simulink model "quick_start_qbot_platform"  (R2023a)
settings: Solver=ode1  StartTime=0.0  StopTime=Inf  FixedStep=1/60  RelTol=1e-3
PostLoadFcn:
  | qlabs_setup
model workspace (MAT data in the model file):
  Sig = Simulink.Signal
  Sig.DataType = 'auto'
  Sig.Dimensions = -1
  Sig.DimensionsMode = 'auto'
  Sig.Complexity = 'auto'
  Sig.SampleTime = -1
  Sig.SamplingMode = 'auto'
  downCamStepSize = Simulink.Parameter
  downCamStepSize.Value = Simulink.data.Expression
  downCamStepSize.Value.ExpressionString = "qc_get_step_size*ceil(1/30/qc_get_step_size)"
  downCamStepSize.DataType = 'auto'
  downCamStepSize.Complexity = 'real'
  downCamStepSize.Dimensions = -1
  lidarStepSize = Simulink.Parameter
  lidarStepSize.Value = Simulink.data.Expression
  lidarStepSize.Value.ExpressionString = "qc_get_step_size*ceil(1/5/qc_get_step_size)"
  lidarStepSize.DataType = 'auto'
  lidarStepSize.Complexity = 'real'
  lidarStepSize.Dimensions = -1
  mainStepSize = Simulink.Parameter
  mainStepSize.Value = Simulink.data.Expression
  mainStepSize.Value.ExpressionString = "qc_get_step_size"
  mainStepSize.DataType = 'auto'
  mainStepSize.Complexity = 'real'
  mainStepSize.Dimensions = -1
  mode = Simulink.Parameter
  mode.Value = 1
  mode.Description = '0 - education speeds via wheel speed commands
    | 1 - education speeds via body speed commands
    | 2 - research speeds via wheel speed commands
    | 3 - research speeds via body speed commands'
  mode.DataType = 'auto'
  mode.Complexity = 'real'
  mode.Dimensions = [1 1]
  realSenseStepSize = Simulink.Parameter
  realSenseStepSize.Value = Simulink.data.Expression
  realSenseStepSize.Value.ExpressionString = "qc_get_step_size*ceil(1/30/qc_get_step_size)"
  realSenseStepSize.DataType = 'auto'
  realSenseStepSize.Complexity = 'real'
  realSenseStepSize.Dimensions = -1
undefined symbols (not defined in the file or in its folder): gcbh, JPEG, Point, qc_get_step_size, Video3D, video_display_show
libraries: quarc_library x31
settings Model: SimulationMode=external  ExtModeTrigDuration=10000  Creator=mbohra  LastModifiedBy=mbohra
settings DebuggingCC: UnderspecifiedInitializationDetection=Classic  MergeDetectMultiDrivingBlocksExec=none
settings ModelReferenceCC: PropagateSignalLabelsOutOfModel=off

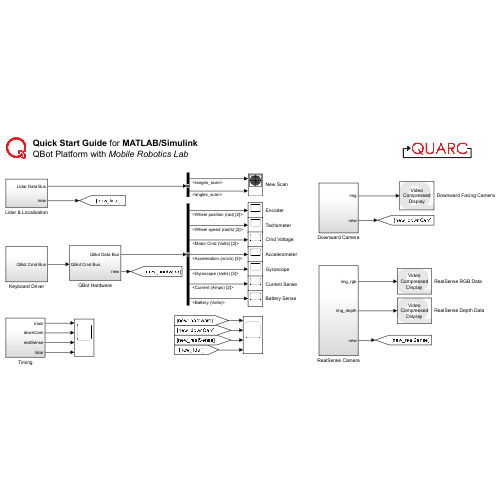
[thumbnail: Simulink's stored preview of the top-level diagram]
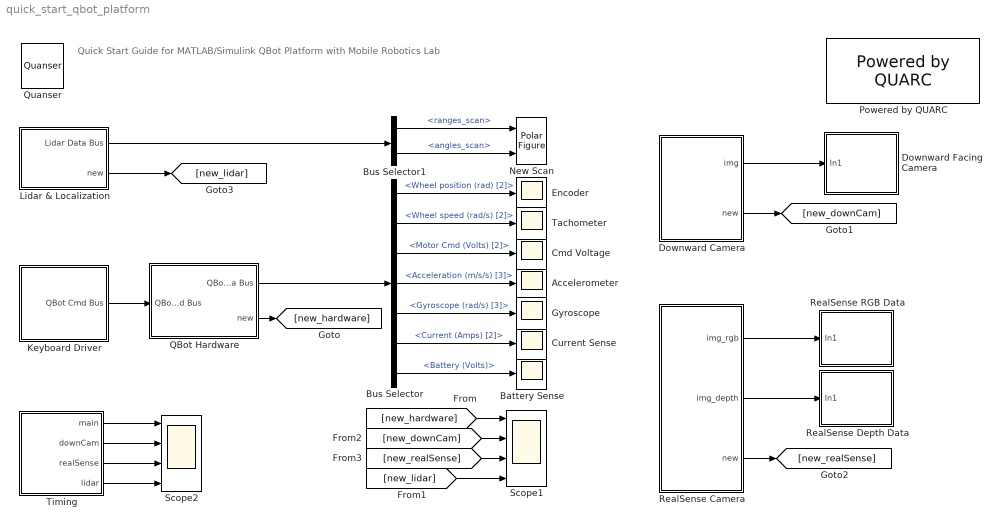
== system quick_start_qbot_platform ==
  note: Quick Start Guide for MATLAB/Simulink
      | QBot Platform with Mobile Robotics Lab
  Accelerometer : Scope
  Battery Sense : Scope
  Bus Selector : BusSelector  OutputSignals=Wheel position (rad) [2],Wheel speed (rad/s) [2],Motor Cmd (Volts) [2],Acceleration (m/s/s) [3],Gyroscope (rad/s) [3],Current (Amps) [2],Battery (Volts)
  Bus Selector1 : BusSelector  OutputSignals=ranges_scan,angles_scan
  Cmd Voltage : Scope
  Current Sense : Scope
  Downward Camera : Subsystem
  Downward Facing Camera : Subsystem  LoadFcn=set_param(gcbh, 'UserData', gcb);  StartFcn=video_display_show([gcb, '/Video Display'], 'add', gcb);  mask(Video Compressed Display){algorithm=JPEG, quality=50, sample_time=-1, use_hardware=on}
      mask prompts: algorithm "Compression algorithm:"; quality "Compression quality (0-100):"; sample_time "Sample time (seconds):"; use_hardware "Use hardware acceleration for video display"
      mask help: Displays a video stream on the host, using compression to minimize bandwidth.
      mask init:
      | qc_set_display('Video\nCompressed\nDisplay');
      settings: UndoDeleteFcn=set_param(gcbh, 'UserData', gcb);  OpenFcn=video_display_show([gcb, '/Video Display'], 'show', gcb);  PreDeleteFcn=video_display_show([gcb, '/Video Display'], 'delete');
      settings: CopyFcn=|
      | set_param(gcbh, 'UserData', gcb);
      | set_param(gcbh, 'LinkStatus', 'none');
      settings: NameChangeFcn=|
      | video_display_show([get_param(gcbh, 'UserData'), '/Video Display'], 'rename', [gcb, '/Video Display']);
      | video_display_show([gcb, '/Video Display'], 'add', gcb);
      | set_param(gcbh, 'UserData', gcb);
      mask Help: web(qc_get_block_help_path(gcb));
      mask TypeOptions algorithm: Image Compress/algorithm
      mask TypeOptions quality: Image Compress/quality
      mask TypeOptions sample_time: Video Display/sample_time
      mask TypeOptions use_hardware: Video Display/use_hardware
      mask Display:
      | patch([0.98591 0.98591 0.62618 0.59072 0.56147   0.536   0.536  0.5441 0.56912 0.59207 0.60881 0.62276 0.63527 0.64364  0.6485  0.6485 0.64706 0.64499 0.63662 0.62411 0.61232 0.59837 0.58307 0.56147   0.536   0.536  0.5441  0.5747 0.60953 0.63662 0.67001  0.7034 0.72851 0.75425 0.77927 0.80294 0.82454 0.84119 0.85865 0.87395 0.88574 0.89339  0.8969 0.89969 0.89969 0.89267  0.8816 0.87044 0.85649  0.8384 0.81824 0.80294 0.78764 0.77513 0.76676 0.75776 0.76397 0.77513 0.79178 0.80987 0.82796 0.84326 0.86207 0.98528],[0.18689 0.05522 0.05522 0.05171 0.05171    0.05 0.18338 0.18338 0.19148 0.20435 0.22298 0.24863 0.28589 0.33125 0.38138 0.55139 0.59801 0.63761 0.68189 0.72149 0.74939 0.76694 0.77855 0.79367 0.79952 0.92768 0.92768 0.92768 0.92417 0.92066 0.91364  0.9032 0.89384 0.88106 0.86594 0.85073 0.82634 0.80537 0.77855 0.74363 0.70403 0.65858 0.61079 0.59099 0.41513 0.37202 0.31847 0.29048 0.25556 0.23342  0.2102 0.19382 0.18221 0.17285 0.16943 0.16124  0.1589 0.16241 0.16709 0.17168  0.1787 0.18221 0.18689 0.18689],[0.9,0.90,0.91])
      | patch([0.536 0.52601 0.46823 0.44528 0.41603 0.39101 0.35555 0.33116 0.31451 0.29291  0.2804 0.26717 0.25322 0.23999 0.22406 0.20732 0.19337 0.17528 0.15935 0.14396 0.13217 0.11759 0.10922 0.10085 0.09671 0.09392 0.09041 0.08906 0.08906 0.09464  0.0995 0.10778 0.11894 0.13145 0.14675 0.16349 0.17672 0.19409 0.20732 0.22406 0.23999 0.26159 0.27833 0.29849 0.31793 0.33602 0.35411 0.37085 0.39245 0.41603   0.536   0.536 0.53159 0.46409   0.446 0.42026 0.39587 0.37571 0.36113 0.34925 0.34088 0.33809 0.33809 0.34088 0.34583 0.35627 0.36392 0.38129 0.39587 0.41117 0.42719 0.44672  0.4676 0.48353 0.48353 0.52394   0.536],[0.05 0.04829 0.04712 0.04712 0.04829 0.05063 0.05405 0.05873 0.06107 0.06692 0.07043 0.07619 0.08087 0.08672 0.09482 0.10652 0.11696 0.13325  0.1508 0.17168 0.19499 0.22415 0.25439 0.28472 0.31379 0.35456 0.38489 0.41513 0.58055 0.63878 0.68774 0.72149 0.75641 0.78089 0.80537 0.82859 0.84029 0.85658 0.86594 0.87404  0.8834 0.89267 0.90086 0.90788 0.91247 0.91832 0.92066   0.923 0.92651 0.92768 0.92768 0.79952 0.79952 0.79952 0.79718 0.78899 0.77153 0.75056 0.72149 0.68072 0.62249  0.5549 0.41396 0.37085 0.33242 0.28121 0.25205 0.22181 0.20552 0.19499 0.18572 0.18221 0.17753 0.17636 0.17753  0.1787  0.1787],[0.9,0.90,0.91])
      | disp('Video\nCompressed\nDisplay');
  Encoder : Scope
  Gyroscope : Scope
  Keyboard Driver : Subsystem
  Lidar & Localization : Subsystem
  New Scan : quarc_library/Sinks/Figures/Polar Figure  figure_mode=Use figure window  figure_tag=figure1  axes_tag=axes1  plot_mode=Frame-based  minimum_rho=0  maximum_rho=4  minimum_theta=0  maximum_theta=360  zero_location=top  direction=counterclockwise  buffer_size=1  update_rate=1  sample_time=-1  initial_position="1340   385   433   389"  initial_visibility=off  line1_style=None  line1_width=0.5  line1_color=[0 0.4470 0.7410]  marker1=Point (.)  marker1_size=6  marker1_edge_color=[0 0.447059 0.741176]  marker1_face_color=[0 0.447059 0.741176]  line2_style=Solid line (-)  line2_width=0.5  line2_color=[0.85098 0.32549 0.0980392]  marker2=None  marker2_size=6  marker2_edge_color=[0.85098 0.32549 0.0980392]  marker2_face_color=[0.85098 0.32549 0.0980392]  line3_style=Solid line (-)  line3_width=0.5  line3_color=[0.929412 0.694118 0.12549]  marker3=None  marker3_size=6  marker3_edge_color=[0.929412 0.694118 0.12549]  marker3_face_color=[0.929412 0.694118 0.12549]  line4_style=Solid line (-)  line4_width=0.5  line4_color=[0.494118 0.184314 0.556863]  marker4=None  marker4_size=6  marker4_edge_color=[0.494118 0.184314 0.556863]  marker4_face_color=[0.494118 0.184314 0.556863]  line5_style=Solid line (-)  line5_width=0.5  line5_color=[0.466667 0.67451 0.188235]  marker5=None  marker5_size=6  marker5_edge_color=[0.466667 0.67451 0.188235]  marker5_face_color=[0.466667 0.67451 0.188235]
      settings: SourceProductName=QUARC Targets
  Powered by QUARC : quarc_library/Logos/Powered by QUARC
  QBot Hardware : Subsystem
  Quanser : quarc_library/Logos/Quanser
  RealSense Camera : Subsystem
  RealSense Depth Data : Subsystem  LoadFcn=set_param(gcbh, 'UserData', gcb);  StartFcn=video_display_show([gcb, '/Video Display'], 'add', gcb);  mask(Video Compressed Display){algorithm=JPEG, quality=50, sample_time=-1, use_hardware=on}
      mask prompts: algorithm "Compression algorithm:"; quality "Compression quality (0-100):"; sample_time "Sample time (seconds):"; use_hardware "Use hardware acceleration for video display"
      mask help: Displays a video stream on the host, using compression to minimize bandwidth.
      mask init:
      | qc_set_display('Video\nCompressed\nDisplay');
      settings: UndoDeleteFcn=set_param(gcbh, 'UserData', gcb);  OpenFcn=video_display_show([gcb, '/Video Display'], 'show', gcb);  PreDeleteFcn=video_display_show([gcb, '/Video Display'], 'delete');
      settings: CopyFcn=|
      | set_param(gcbh, 'UserData', gcb);
      | set_param(gcbh, 'LinkStatus', 'none');
      settings: NameChangeFcn=|
      | video_display_show([get_param(gcbh, 'UserData'), '/Video Display'], 'rename', [gcb, '/Video Display']);
      | video_display_show([gcb, '/Video Display'], 'add', gcb);
      | set_param(gcbh, 'UserData', gcb);
      mask Help: web(qc_get_block_help_path(gcb));
      mask TypeOptions algorithm: Image Compress/algorithm
      mask TypeOptions quality: Image Compress/quality
      mask TypeOptions sample_time: Video Display/sample_time
      mask TypeOptions use_hardware: Video Display/use_hardware
      mask Display:
      | patch([0.98591 0.98591 0.62618 0.59072 0.56147   0.536   0.536  0.5441 0.56912 0.59207 0.60881 0.62276 0.63527 0.64364  0.6485  0.6485 0.64706 0.64499 0.63662 0.62411 0.61232 0.59837 0.58307 0.56147   0.536   0.536  0.5441  0.5747 0.60953 0.63662 0.67001  0.7034 0.72851 0.75425 0.77927 0.80294 0.82454 0.84119 0.85865 0.87395 0.88574 0.89339  0.8969 0.89969 0.89969 0.89267  0.8816 0.87044 0.85649  0.8384 0.81824 0.80294 0.78764 0.77513 0.76676 0.75776 0.76397 0.77513 0.79178 0.80987 0.82796 0.84326 0.86207 0.98528],[0.18689 0.05522 0.05522 0.05171 0.05171    0.05 0.18338 0.18338 0.19148 0.20435 0.22298 0.24863 0.28589 0.33125 0.38138 0.55139 0.59801 0.63761 0.68189 0.72149 0.74939 0.76694 0.77855 0.79367 0.79952 0.92768 0.92768 0.92768 0.92417 0.92066 0.91364  0.9032 0.89384 0.88106 0.86594 0.85073 0.82634 0.80537 0.77855 0.74363 0.70403 0.65858 0.61079 0.59099 0.41513 0.37202 0.31847 0.29048 0.25556 0.23342  0.2102 0.19382 0.18221 0.17285 0.16943 0.16124  0.1589 0.16241 0.16709 0.17168  0.1787 0.18221 0.18689 0.18689],[0.9,0.90,0.91])
      | patch([0.536 0.52601 0.46823 0.44528 0.41603 0.39101 0.35555 0.33116 0.31451 0.29291  0.2804 0.26717 0.25322 0.23999 0.22406 0.20732 0.19337 0.17528 0.15935 0.14396 0.13217 0.11759 0.10922 0.10085 0.09671 0.09392 0.09041 0.08906 0.08906 0.09464  0.0995 0.10778 0.11894 0.13145 0.14675 0.16349 0.17672 0.19409 0.20732 0.22406 0.23999 0.26159 0.27833 0.29849 0.31793 0.33602 0.35411 0.37085 0.39245 0.41603   0.536   0.536 0.53159 0.46409   0.446 0.42026 0.39587 0.37571 0.36113 0.34925 0.34088 0.33809 0.33809 0.34088 0.34583 0.35627 0.36392 0.38129 0.39587 0.41117 0.42719 0.44672  0.4676 0.48353 0.48353 0.52394   0.536],[0.05 0.04829 0.04712 0.04712 0.04829 0.05063 0.05405 0.05873 0.06107 0.06692 0.07043 0.07619 0.08087 0.08672 0.09482 0.10652 0.11696 0.13325  0.1508 0.17168 0.19499 0.22415 0.25439 0.28472 0.31379 0.35456 0.38489 0.41513 0.58055 0.63878 0.68774 0.72149 0.75641 0.78089 0.80537 0.82859 0.84029 0.85658 0.86594 0.87404  0.8834 0.89267 0.90086 0.90788 0.91247 0.91832 0.92066   0.923 0.92651 0.92768 0.92768 0.79952 0.79952 0.79952 0.79718 0.78899 0.77153 0.75056 0.72149 0.68072 0.62249  0.5549 0.41396 0.37085 0.33242 0.28121 0.25205 0.22181 0.20552 0.19499 0.18572 0.18221 0.17753 0.17636 0.17753  0.1787  0.1787],[0.9,0.90,0.91])
      | disp('Video\nCompressed\nDisplay');
  RealSense RGB Data : Subsystem  LoadFcn=set_param(gcbh, 'UserData', gcb);  StartFcn=video_display_show([gcb, '/Video Display'], 'add', gcb);  mask(Video Compressed Display){algorithm=JPEG, quality=50, sample_time=-1, use_hardware=on}
      mask prompts: algorithm "Compression algorithm:"; quality "Compression quality (0-100):"; sample_time "Sample time (seconds):"; use_hardware "Use hardware acceleration for video display"
      mask help: Displays a video stream on the host, using compression to minimize bandwidth.
      mask init:
      | qc_set_display('Video\nCompressed\nDisplay');
      settings: UndoDeleteFcn=set_param(gcbh, 'UserData', gcb);  OpenFcn=video_display_show([gcb, '/Video Display'], 'show', gcb);  PreDeleteFcn=video_display_show([gcb, '/Video Display'], 'delete');
      settings: CopyFcn=|
      | set_param(gcbh, 'UserData', gcb);
      | set_param(gcbh, 'LinkStatus', 'none');
      settings: NameChangeFcn=|
      | video_display_show([get_param(gcbh, 'UserData'), '/Video Display'], 'rename', [gcb, '/Video Display']);
      | video_display_show([gcb, '/Video Display'], 'add', gcb);
      | set_param(gcbh, 'UserData', gcb);
      mask Help: web(qc_get_block_help_path(gcb));
      mask TypeOptions algorithm: Image Compress/algorithm
      mask TypeOptions quality: Image Compress/quality
      mask TypeOptions sample_time: Video Display/sample_time
      mask TypeOptions use_hardware: Video Display/use_hardware
      mask Display:
      | patch([0.98591 0.98591 0.62618 0.59072 0.56147   0.536   0.536  0.5441 0.56912 0.59207 0.60881 0.62276 0.63527 0.64364  0.6485  0.6485 0.64706 0.64499 0.63662 0.62411 0.61232 0.59837 0.58307 0.56147   0.536   0.536  0.5441  0.5747 0.60953 0.63662 0.67001  0.7034 0.72851 0.75425 0.77927 0.80294 0.82454 0.84119 0.85865 0.87395 0.88574 0.89339  0.8969 0.89969 0.89969 0.89267  0.8816 0.87044 0.85649  0.8384 0.81824 0.80294 0.78764 0.77513 0.76676 0.75776 0.76397 0.77513 0.79178 0.80987 0.82796 0.84326 0.86207 0.98528],[0.18689 0.05522 0.05522 0.05171 0.05171    0.05 0.18338 0.18338 0.19148 0.20435 0.22298 0.24863 0.28589 0.33125 0.38138 0.55139 0.59801 0.63761 0.68189 0.72149 0.74939 0.76694 0.77855 0.79367 0.79952 0.92768 0.92768 0.92768 0.92417 0.92066 0.91364  0.9032 0.89384 0.88106 0.86594 0.85073 0.82634 0.80537 0.77855 0.74363 0.70403 0.65858 0.61079 0.59099 0.41513 0.37202 0.31847 0.29048 0.25556 0.23342  0.2102 0.19382 0.18221 0.17285 0.16943 0.16124  0.1589 0.16241 0.16709 0.17168  0.1787 0.18221 0.18689 0.18689],[0.9,0.90,0.91])
      | patch([0.536 0.52601 0.46823 0.44528 0.41603 0.39101 0.35555 0.33116 0.31451 0.29291  0.2804 0.26717 0.25322 0.23999 0.22406 0.20732 0.19337 0.17528 0.15935 0.14396 0.13217 0.11759 0.10922 0.10085 0.09671 0.09392 0.09041 0.08906 0.08906 0.09464  0.0995 0.10778 0.11894 0.13145 0.14675 0.16349 0.17672 0.19409 0.20732 0.22406 0.23999 0.26159 0.27833 0.29849 0.31793 0.33602 0.35411 0.37085 0.39245 0.41603   0.536   0.536 0.53159 0.46409   0.446 0.42026 0.39587 0.37571 0.36113 0.34925 0.34088 0.33809 0.33809 0.34088 0.34583 0.35627 0.36392 0.38129 0.39587 0.41117 0.42719 0.44672  0.4676 0.48353 0.48353 0.52394   0.536],[0.05 0.04829 0.04712 0.04712 0.04829 0.05063 0.05405 0.05873 0.06107 0.06692 0.07043 0.07619 0.08087 0.08672 0.09482 0.10652 0.11696 0.13325  0.1508 0.17168 0.19499 0.22415 0.25439 0.28472 0.31379 0.35456 0.38489 0.41513 0.58055 0.63878 0.68774 0.72149 0.75641 0.78089 0.80537 0.82859 0.84029 0.85658 0.86594 0.87404  0.8834 0.89267 0.90086 0.90788 0.91247 0.91832 0.92066   0.923 0.92651 0.92768 0.92768 0.79952 0.79952 0.79952 0.79718 0.78899 0.77153 0.75056 0.72149 0.68072 0.62249  0.5549 0.41396 0.37085 0.33242 0.28121 0.25205 0.22181 0.20552 0.19499 0.18572 0.18221 0.17753 0.17636 0.17753  0.1787  0.1787],[0.9,0.90,0.91])
      | disp('Video\nCompressed\nDisplay');
  Scope1 : Scope  NumInputPorts=4
  Scope2 : Scope  NumInputPorts=4
  Tachometer : Scope
  Timing : Subsystem
  wires:
  Timing/1(main) -> Scope2/1
  Timing/2(downCam) -> Scope2/2
  Timing/3(realSense) -> Scope2/3
  Timing/4(lidar) -> Scope2/4
  Lidar & Localization/1(Lidar Data Bus) -> Bus Selector1/1
  QBot Hardware/1(QBot Data Bus) -> Bus Selector/1
  QBot Hardware/2(new) -> [new_hardware]
  Lidar & Localization/2(new) -> [new_lidar]
  Downward Camera/2(new) -> [new_downCam]
  RealSense Camera/3(new) -> [new_realSense]
  [new_hardware] -> Scope1/1
  [new_realSense] -> Scope1/3
  [new_lidar] -> Scope1/4
  [new_downCam] -> Scope1/2
  Bus Selector/1 -> Encoder/1  "<Wheel position (rad) [2]>"
  Bus Selector/3 -> Cmd Voltage/1  "<Motor Cmd (Volts) [2]>"
  Bus Selector/4 -> Accelerometer/1  "<Acceleration (m/s/s) [3]>"
  Bus Selector/6 -> Current Sense/1  "<Current (Amps) [2]>"
  Bus Selector/2 -> Tachometer/1  "<Wheel speed (rad/s) [2]>"
  Bus Selector/5 -> Gyroscope/1  "<Gyroscope (rad/s) [3]>"
  Bus Selector/7 -> Battery Sense/1  "<Battery (Volts)>"
  Bus Selector1/1 -> New Scan/1  "<ranges_scan>"
  Bus Selector1/2 -> New Scan/2  "<angles_scan>"
  Downward Camera/1(img) -> Downward Facing Camera/1(In1)
  RealSense Camera/2(img_depth) -> RealSense Depth Data/1(In1)
  RealSense Camera/1(img_rgb) -> RealSense RGB Data/1(In1)
  Keyboard Driver/1(QBot Cmd Bus) -> QBot Hardware/1(QBot Cmd Bus)

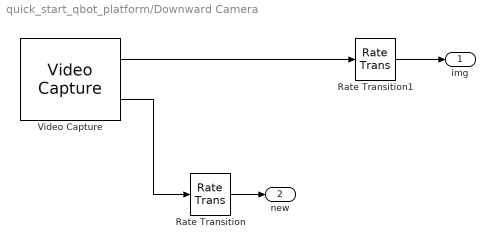
== system quick_start_qbot_platform/Downward Camera ==
  Rate Transition : RateTransition
  Rate Transition1 : RateTransition  OutPortSampleTime=downCamStepSize*4
  Video Capture : quarc_library/Multimedia/Video Capture  source=device  device=0@tcpip://localhost:18915  filename=sample_movie.mov  value=[0 0; 0 0]  resolution=640 x 400  width=640  height=400  output_format=MATLAB greyscale (HxW)  data_type=uint8  sample_time=downCamStepSize  brightness_override=off  brightness=50.0  contrast_override=off  contrast=50.0  hue_override=off  hue=50.0  saturation_override=off  saturation=50.0  sharpness_override=off  sharpness=50.0  gamma_override=off  gamma=50.0  coloreffect_override=off  coloreffect=None  whitebalance_override=off  whitebalance=50.0  backlightcompensation_override=off  backlightcompensation=0.0  gain_override=on  gain=27.0  pan_override=off  pan=50.0  tilt_override=off  tilt=50.0  roll_override=off  roll=50.0  zoom_override=off  zoom=0.0  exposure_override=on  exposure=60.0  iris_override=off  iris=50.0  mirror_override=off  mirror=None  focus_override=off  focus=0.0
      settings: SourceProductName=QUARC Targets
  img : Outport
  new : Outport  Port=2
  wires:
  Video Capture/2 -> Rate Transition/1
  Video Capture/1 -> Rate Transition1/1
  Rate Transition/1 -> new/1
  Rate Transition1/1 -> img/1

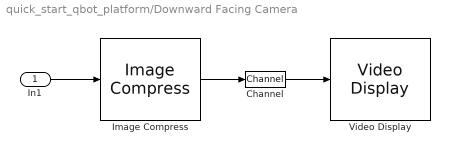
== system quick_start_qbot_platform/Downward Facing Camera ==
  In1 : Inport
  Channel : quarc_library/Signal Routing/Channel  channel=0  buffer_size=1
  Image Compress : quarc_library/Image Processing/Generic/Image Compress  algorithm=JPEG  source=Internal dialog parameter  quality=quality  output_dim=-1
  Video Display : quarc_library/Multimedia/Video Display  Tag=quick_start_qbot_platform_t/Downward Facing Camera/Video Display  sample_time=sample_time  use_hardware=on
  wires:
  Image Compress/1 -> Channel/1
  In1/1 -> Image Compress/1
  Channel/1 -> Video Display/1

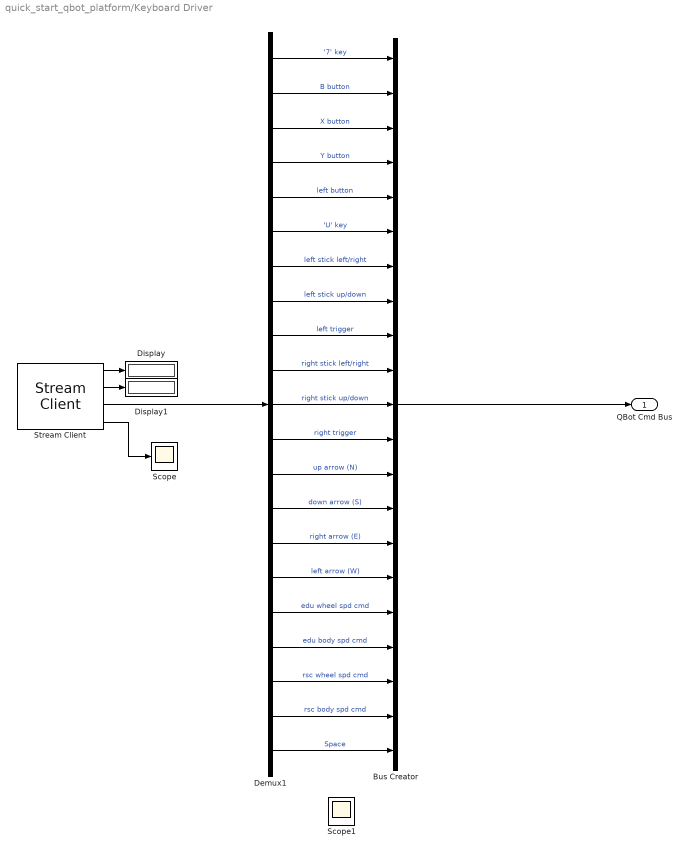
== system quick_start_qbot_platform/Keyboard Driver ==
  Bus Creator : BusCreator  Inputs=21
  Demux1 : Demux  Outputs=[1 1 1 1 1 1 1 1 1 1 1 1 1 1 1 1 2 2 2 2 1]
  Display : Display
  Display1 : Display
  Scope : Scope
  Scope1 : Scope
  Stream Client : quarc_library/Communications/Basic/Stream Client  uri_source=Specify via dialog (do not evaluate)  uri=tcpip://localhost:18889?nagle='off'  send_buffer_size=1460  receive_buffer_size=1460  byte_order=little endian (Intel - LSB first)  optimization=Minimum latency  send_options=Do not send data  receive_options=Receive most recent data  default_value=zeros(25,1)  sample_time=qc_get_step_size  active=on  implementation=Use blocking I/O in a separate thread  send_fifo_size=1000  receive_fifo_size=1000  send_priority=0  receive_priority=0  send_dimensions=off  receive_dimensions=off  max_dimensions=-1  data_type=Inherited via back propagation  type_expr=BusObject
      settings: AttributesFormatString="\"tcpip://localhost:18889?nagle='off'\""
  QBot Cmd Bus : Outport
  wires:
  Bus Creator/1 -> QBot Cmd Bus/1
  Stream Client/3 -> Demux1/1
  Demux1/1 -> Bus Creator/1  "'7' key"
  Demux1/2 -> Bus Creator/2  "B button"
  Demux1/3 -> Bus Creator/3  "X button"
  Demux1/4 -> Bus Creator/4  "Y button"
  Demux1/5 -> Bus Creator/5  "left button"
  Demux1/6 -> Bus Creator/6  "'U' key"
  Demux1/7 -> Bus Creator/7  "left stick left/right"
  Demux1/8 -> Bus Creator/8  "left stick up/down"
  Demux1/9 -> Bus Creator/9  "left trigger"
  Demux1/10 -> Bus Creator/10  "right stick left/right"
  Demux1/11 -> Bus Creator/11  "right stick up/down"
  Demux1/12 -> Bus Creator/12  "right trigger"
  Demux1/13 -> Bus Creator/13  "up arrow (N)"
  Demux1/14 -> Bus Creator/14  "down arrow (S)"
  Demux1/15 -> Bus Creator/15  "right arrow (E)"
  Demux1/16 -> Bus Creator/16  "left arrow (W)"
  Demux1/17 -> Bus Creator/17  "edu wheel spd cmd"
  Demux1/18 -> Bus Creator/18  "edu body spd cmd"
  Demux1/19 -> Bus Creator/19  "rsc wheel spd cmd"
  Demux1/20 -> Bus Creator/20  "rsc body spd cmd"
  Demux1/21 -> Bus Creator/21  "Space"
  Stream Client/1 -> Display/1
  Stream Client/2 -> Display1/1
  Stream Client/4 -> Scope/1

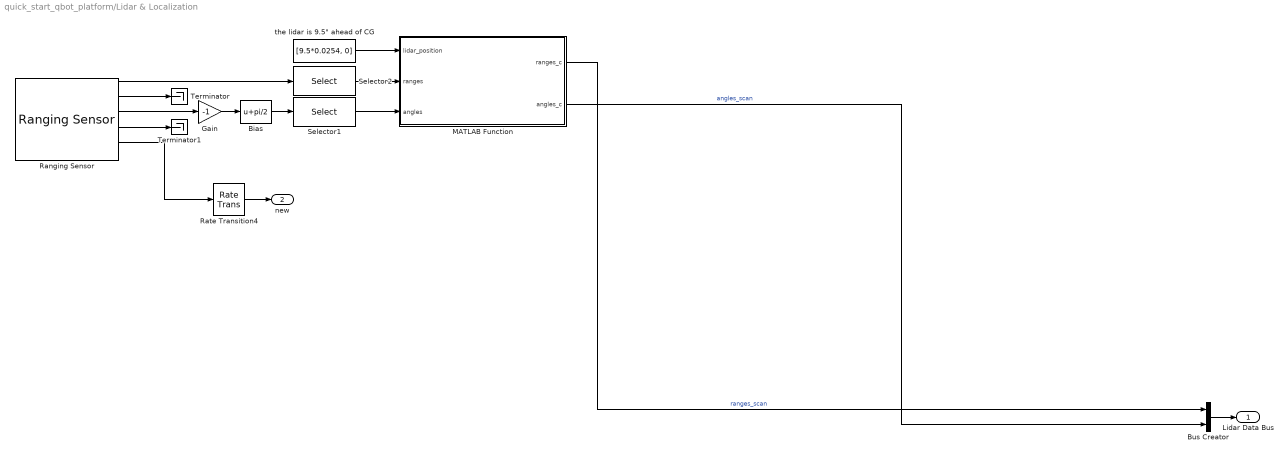
== system quick_start_qbot_platform/Lidar & Localization ==
  Bias : Bias  Bias=pi/2  SaturateOnIntegerOverflow=off
  Bus Creator : BusCreator  Inputs=2
  Gain : Gain  Gain=-1
  MATLAB Function : MATLAB Function  TreatAsAtomicUnit=on
  Ranging Sensor : quarc_library/Devices/Third-Party/Sensors/Ranging Sensor  sensor_type=Leishen M10P LIDAR  uri=tcpip://localhost:18918  ranging_distance=Short  timing_budget=0.033  measurement_period=0.0005  output_mode=Fixed-size output  samples_per_revolution=1680  max_distance=0.050  max_angle=5  sample_time=lidarStepSize  show_versions=off  active=on
      settings: SourceProductName=QUARC Targets
  Rate Transition4 : RateTransition
  Selector1 : Selector  InputPortWidth=1680  IndexOptions=Index vector (dialog)  Indices=[1:4:1677]  OutputSizes=1
  Selector2 : Selector  InputPortWidth=1680  IndexOptions=Index vector (dialog)  Indices=[1:4:1677]  OutputSizes=1
  Terminator : Terminator
  Terminator1 : Terminator
  "the lidar is 9.5\" ahead of CG" : Constant  Value=[9.5*0.0254, 0]  SampleTime=lidarStepSize
  Lidar Data Bus : Outport
  new : Outport  Port=2
  wires:
  Ranging Sensor/5 -> Rate Transition4/1
  Rate Transition4/1 -> new/1
  Selector1/1 -> MATLAB Function/3(angles)
  Selector2/1 -> MATLAB Function/2(ranges)
  "the lidar is 9.5\" ahead of CG"/1 -> MATLAB Function/1(lidar_position)
  Bias/1 -> Selector1/1
  Ranging Sensor/2 -> Terminator/1
  Ranging Sensor/4 -> Terminator1/1
  Gain/1 -> Bias/1
  Ranging Sensor/3 -> Gain/1
  Ranging Sensor/1 -> Selector2/1
  MATLAB Function/1(ranges_c) -> Bus Creator/1  "ranges_scan"
  MATLAB Function/2(angles_c) -> Bus Creator/2  "angles_scan"
  Bus Creator/1 -> Lidar Data Bus/1

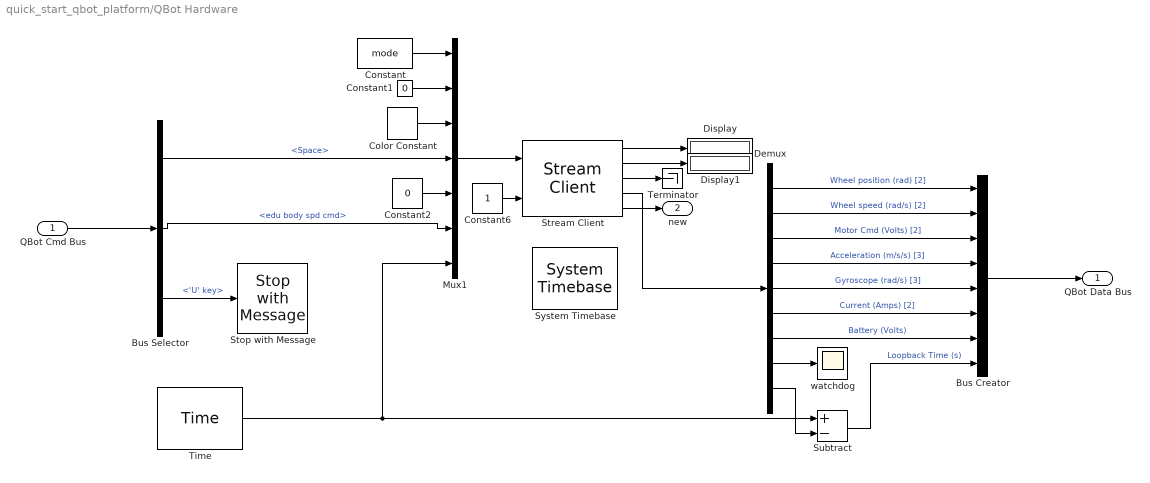
== system quick_start_qbot_platform/QBot Hardware ==
  QBot Cmd Bus : Inport
  Bus Creator : BusCreator  Inputs=8
  Bus Selector : BusSelector  OutputSignals=Space,edu body spd cmd,'U' key
  Color Constant : quarc_library/Sources/Signals/Color Constant  color=[0 1 1]
      settings: SourceProductName=QUARC Targets
  Constant : Constant  Value=mode
  Constant1 : Constant  Value=0
  Constant2 : Constant  Value=0
  Constant6 : Constant
  Demux : Demux  Outputs=[2 2 2 3 3 2 1 1 1]
  Display : Display
  Display1 : Display
  Mux1 : Mux  Inputs=7
  Stop with Message : quarc_library/Sinks/Error Handling/Stop with Message  message_type=Fixed error message  message_icon=Information  message=Operator: Emergency Stop
  Stream Client : quarc_library/Communications/Basic/Stream Client  uri_source=Specify via dialog (do not evaluate)  uri=tcpip://localhost:18888  send_buffer_size=1460  receive_buffer_size=1460  byte_order=little endian (Intel - LSB first)  optimization=Minimum latency  send_options=Send most recent data  receive_options=Receive most recent data  default_value=zeros(17,1)  sample_time=qc_get_step_size  active=on  implementation=Use blocking I/O in a separate thread  send_fifo_size=1000  receive_fifo_size=1000  send_priority=0  receive_priority=0  send_dimensions=off  receive_dimensions=off  max_dimensions=-1  data_type=Inherited via back propagation  type_expr=BusObject
      settings: AttributesFormatString="\"tcpip://localhost:18888\""
  Subtract : Sum  Inputs=+-
  System Timebase : quarc_library/Advanced/Timing/System Timebase  stop_on_overrun=off
      settings: SourceProductName=QUARC Targets
  Terminator : Terminator
  Time : quarc_library/Sources/Time/Time  time_source=Wall clock  sample_time=qc_get_step_size
  watchdog : Scope
  QBot Data Bus : Outport
  new : Outport  Port=2
  wires:
  Demux/2 -> Bus Creator/2  "Wheel speed (rad/s) [2]"
  Constant/1 -> Mux1/1
  Stream Client/3 -> Terminator/1
  Stream Client/1 -> Display/1
  Constant6/1 -> Stream Client/2
  Stream Client/2 -> Display1/1
  Color Constant/1 -> Mux1/3
  Constant1/1 -> Mux1/2
  Demux/3 -> Bus Creator/3  "Motor Cmd (Volts) [2]"
  Mux1/1 -> Stream Client/1
  Stream Client/4 -> Demux/1
  Demux/1 -> Bus Creator/1  "Wheel position (rad) [2]"
  Stream Client/5 -> new/1
  Demux/7 -> Bus Creator/7  "Battery (Volts)"
  Demux/5 -> Bus Creator/5  "Gyroscope (rad/s) [3]"
  Demux/6 -> Bus Creator/6  "Current (Amps) [2]"
  Demux/9 -> Subtract/2
  Constant2/1 -> Mux1/5
  Demux/4 -> Bus Creator/4  "Acceleration (m/s/s) [3]"
  Time/1 -> Subtract/1, Mux1/7
  Bus Creator/1 -> QBot Data Bus/1
  Subtract/1 -> Bus Creator/8  "Loopback Time (s)"
  Demux/8 -> watchdog/1
  QBot Cmd Bus/1 -> Bus Selector/1
  Bus Selector/3 -> Stop with Message/1  "<'U' key>"
  Bus Selector/2 -> Mux1/6  "<edu body spd cmd>"
  Bus Selector/1 -> Mux1/4  "<Space>"

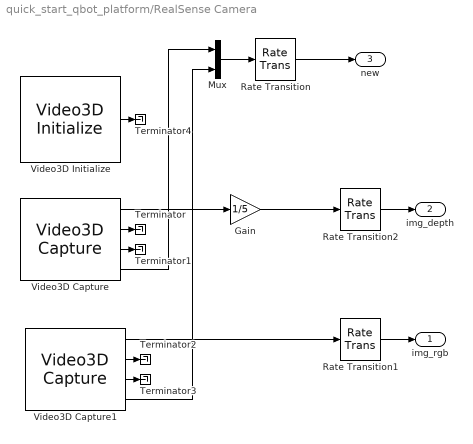
== system quick_start_qbot_platform/RealSense Camera ==
  Gain : Gain  Gain=1/5
  Mux : Mux  Inputs=2
  Rate Transition : RateTransition
  Rate Transition1 : RateTransition  OutPortSampleTime=realSenseStepSize*2
  Rate Transition2 : RateTransition  OutPortSampleTime=realSenseStepSize*2
  Terminator{,1..4} (5 alike) : Terminator
  Video3D Capture : quarc_library/Multimedia/Video3D Capture  object_name=Video3D-1  stream_type=Depth  stream_index=0  resolution=640 x 480  width=640  height=480  output_format=Distance in meters (HxW)  data_type=single  sample_time=realSenseStepSize  camera_intrinsics=off  depth_scale=off  brightness_override=off  brightness=50.0  contrast_override=off  contrast=50.0  hue_override=off  hue=50.0  saturation_override=off  saturation=50.0  sharpness_override=off  sharpness=50.0  gamma_override=off  gamma=50.0  gain_override=off  gain=50.0  backlightcompensation_override=off  backlightcompensation=50.0  whitebalance_override=Automatic white balance  whitebalance=50.0  exposure_override=Automatic exposure  exposure=30.0  emitter=Enable laser emitter  preset=Do not set camera presets
  Video3D Capture1 : quarc_library/Multimedia/Video3D Capture  object_name=Video3D-1  stream_type=RGB  stream_index=0  resolution=640 x 480  width=640  height=480  output_format=MATLAB RGB (HxWx3)  data_type=uint8  sample_time=realSenseStepSize  camera_intrinsics=off  depth_scale=off  brightness_override=off  brightness=50.0  contrast_override=off  contrast=50.0  hue_override=off  hue=50.0  saturation_override=off  saturation=50.0  sharpness_override=off  sharpness=50.0  gamma_override=off  gamma=50.0  gain_override=off  gain=50.0  backlightcompensation_override=off  backlightcompensation=50.0  whitebalance_override=Automatic white balance  whitebalance=50.0  exposure_override=Automatic exposure  exposure=30.0  emitter=Enable laser emitter  preset=Do not set camera presets
  Video3D Initialize : quarc_library/Multimedia/Video3D Initialize  object_name=Video3D-1  source=Device  identifier=0@tcpip://localhost:18917  file=sample.bag  sample_time=qc_get_step_size *2  active=on
  img_rgb : Outport
  img_depth : Outport  Port=2
  new : Outport  Port=3
  wires:
  Video3D Capture1/1 -> Rate Transition1/1
  Mux/1 -> Rate Transition/1
  Video3D Capture/4 -> Mux/1
  Video3D Capture1/4 -> Mux/2
  Video3D Capture/2 -> Terminator/1
  Video3D Capture/3 -> Terminator1/1
  Video3D Capture1/2 -> Terminator2/1
  Video3D Capture1/3 -> Terminator3/1
  Video3D Initialize/1 -> Terminator4/1
  Rate Transition/1 -> new/1
  Rate Transition1/1 -> img_rgb/1
  Rate Transition2/1 -> img_depth/1
  Video3D Capture/1 -> Gain/1
  Gain/1 -> Rate Transition2/1

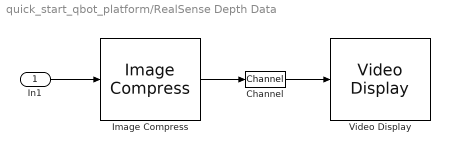
== system quick_start_qbot_platform/RealSense Depth Data ==
  In1 : Inport
  Channel : quarc_library/Signal Routing/Channel  channel=1  buffer_size=1
  Image Compress : quarc_library/Image Processing/Generic/Image Compress  algorithm=JPEG  source=Internal dialog parameter  quality=quality  output_dim=-1
  Video Display : quarc_library/Multimedia/Video Display  Tag=quick_start_qbot_platform_t/RealSense Depth Data/Video Display  sample_time=sample_time  use_hardware=on
  wires:
  Channel/1 -> Video Display/1
  In1/1 -> Image Compress/1
  Image Compress/1 -> Channel/1

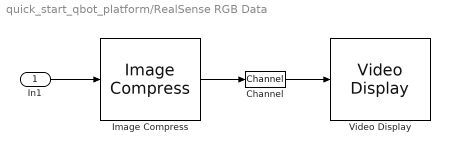
== system quick_start_qbot_platform/RealSense RGB Data ==
  In1 : Inport
  Channel : quarc_library/Signal Routing/Channel  channel=2  buffer_size=1
  Image Compress : quarc_library/Image Processing/Generic/Image Compress  algorithm=JPEG  source=Internal dialog parameter  quality=quality  output_dim=-1
  Video Display : quarc_library/Multimedia/Video Display  Tag=quick_start_qbot_platform_t/RealSense RGB Data/Video Display  sample_time=sample_time  use_hardware=on
  wires:
  Image Compress/1 -> Channel/1
  In1/1 -> Image Compress/1
  Channel/1 -> Video Display/1

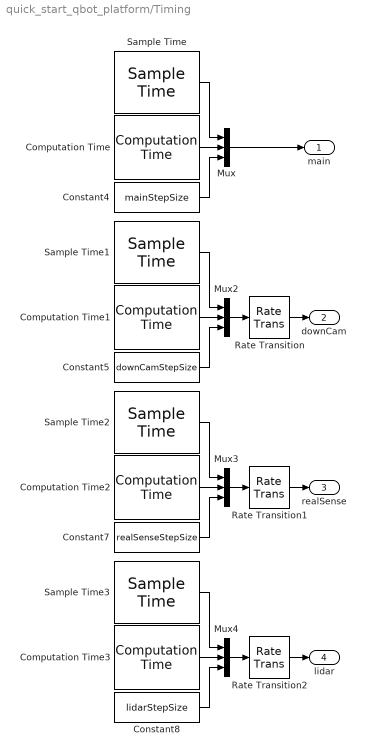
== system quick_start_qbot_platform/Timing ==
  Computation Time : quarc_library/Sources/Time/Computation Time  sample_time=mainStepSize  use_model=on  use_cpu_time=off
  Computation Time1 : quarc_library/Sources/Time/Computation Time  sample_time=downCamStepSize  use_model=on  use_cpu_time=off
  Computation Time2 : quarc_library/Sources/Time/Computation Time  sample_time=realSenseStepSize  use_model=on  use_cpu_time=off
  Computation Time3 : quarc_library/Sources/Time/Computation Time  sample_time=lidarStepSize  use_model=on  use_cpu_time=off
  Constant4 : Constant  Value=mainStepSize
  Constant5 : Constant  Value=downCamStepSize
  Constant7 : Constant  Value=realSenseStepSize
  Constant8 : Constant  Value=lidarStepSize
  Mux{,2..4} (4 alike) : Mux  Inputs=3
  Rate Transition : RateTransition
  Rate Transition1 : RateTransition
  Rate Transition2 : RateTransition
  Sample Time : quarc_library/Sources/Time/Sample Time  Priority=-99  sample_time=mainStepSize
  Sample Time1 : quarc_library/Sources/Time/Sample Time  Priority=-99  sample_time=downCamStepSize
  Sample Time2 : quarc_library/Sources/Time/Sample Time  Priority=-99  sample_time=realSenseStepSize
  Sample Time3 : quarc_library/Sources/Time/Sample Time  Priority=-99  sample_time=lidarStepSize
  main : Outport
  downCam : Outport  Port=2
  realSense : Outport  Port=3
  lidar : Outport  Port=4
  wires:
  Rate Transition1/1 -> realSense/1
  Computation Time2/1 -> Mux3/2
  Constant5/1 -> Mux2/3
  Mux4/1 -> Rate Transition2/1
  Computation Time/1 -> Mux/2
  Sample Time/1 -> Mux/1
  Constant8/1 -> Mux4/3
  Sample Time1/1 -> Mux2/1
  Mux3/1 -> Rate Transition1/1
  Computation Time1/1 -> Mux2/2
  Constant4/1 -> Mux/3
  Mux2/1 -> Rate Transition/1
  Computation Time3/1 -> Mux4/2
  Sample Time2/1 -> Mux3/1
  Constant7/1 -> Mux3/3
  Sample Time3/1 -> Mux4/1
  Rate Transition/1 -> downCam/1
  Rate Transition2/1 -> lidar/1
  Mux/1 -> main/1

== matlab function quick_start_qbot_platform/Lidar & Localization/MATLAB Function ==
  data: lidar_position input; ranges input; ranges_c output; angles input; angles_c output
function [ranges_c,angles_c] = correct_lidar(lidar_position, ranges,angles)

x = ranges.*cos(angles) + lidar_position(1);
y = ranges.*sin(angles) + lidar_position(2);

ranges_c = sqrt(x.^2 + y.^2);
angles_c = atan2(y, x);

end
